simulink model "fuzzyRIP_LQR"  (Simulink 8.1)
settings: Solver=ode45  StartTime=0.0  StopTime=20  RelTol=1e-3
StopFcn:
  | subplot(3,1,1);
  | plot(Data.time, Data.signals(1,1).values,'-r','LineWidth',1.5)
  | legend('alpha');
  | grid;
  | ylabel('alpha [rad]');
  | title ('FuzzyController');
  | subplot(3,1,2);
  | plot(Data.time, Data.signals(1,3).values,'-b','LineWidth',1.5)
  | legend('theta');
  | grid;
  | ylabel('theta [rad]');
  | subplot(3,1,3);
  | plot(Data.time, Data.signals(1,5).values,'-g','LineWidth',1.5)
  | legend('Voltage');
  | grid;
  | ylabel('voltage [V]');
libraries: fuzblock x1
settings Model: Creator=ThanhNhan  LastModifiedBy=ThanhNhan
settings DataIOCC: SignalLoggingSaveFormat=Dataset
settings OptimizationCC: ExpressionDepthLimit=128
settings DebuggingCC: FcnCallInpInsideContextMsg=EnableAllAsError
settings GRTTargetCC: CombineOutputUpdateFcns=on  GRTInterface=off

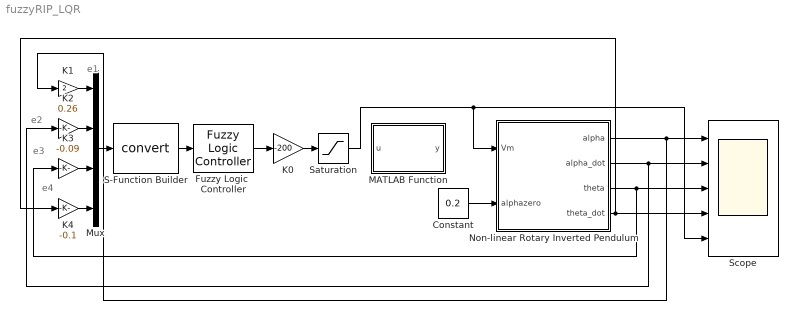
== system fuzzyRIP_LQR ==
  note: e4
  note: e3
  note: e2
  note: e1
  Constant : Constant  Value=0.2
  Fuzzy Logic  Controller : fuzblock/Fuzzy Logic  Controller  fis='RIPfuzzyMam5.fis'
  K0 : Gain  Gain=-200
  K1 : Gain  Gain=2
  K2 : Gain  Gain=0.26
  K3 : Gain  Gain=-0.09
  K4 : Gain  Gain=-0.1
  MATLAB Function : MATLAB Function  TreatAsAtomicUnit=on
  Mux : Mux
  Non-linear Rotary Inverted Pendulum : Subsystem  mask{Jeq=0.004036, g=9.81, m=0.05562, L=0.1254, r=0.1095, Beq=0.0444, eta=0.69, Km=0.084026, Kt=0.084039, Rm=2.6, Jm=0.001}
      mask prompts: Jeq "Momen quán tính tuong duong (Jeq)"; g "Gia toc trong truong (g)"; m "Khoi luong con lac (m)"; L "Nua chieu dai con lac (L)"; r "Nua chieu dài cánh tay (r)"; Beq "He so can tuong duong (Beq)"; eta "Hieu suat dong co (eta)"; Km "Hang so suc dien dong (Km)"; Kt "Hang so momen  (Kt)"; Rm "Dien tro phan ung (Rm)"; Jm "Momen quan tinh dong co (Jm)"
  S-Function Builder : S-Function  InitFcn=try, set_param(gcb,'FunctionName','convert'), end  FunctionName=convert  SFunctionModules=convert_wrapper  WizardData=DataTag0  EnableBusSupport=off  mask(S-Function Builder){}
      mask help: Simulink:masks:SFunctionBuilder_MD
      mask init:
      | val = [[.9  0.75 0.75 1 1 .9 .9 1]',[1 1 0.75 0.75 .9 .9 1 .9]'];try , sys = get_param(gcb,'SfunBuilderFcnName');if isempty(sys), sys = get_param(gcb,'FunctionName'); end,catch, sys = get_param(gcb,'FunctionName'); end
      settings: CopyFcn=set_param(gcbh,'LinkStatus','none')  PreSaveFcn=try, set_param(gcb,'FunctionName','convert'), end  OpenFcn=sfunctionwizard(gcbh)
      mask Display: plot(val(:,1),val(:,2)),disp(sys), port_label('input',1,'u0'), port_label('output',1,'y0')
  Saturation : Saturate  UpperLimit=24  LowerLimit=-24
  Scope : Scope  NumInputPorts=5
      settings: YMin=-29.91~-1500~5e+07~1e+08~-5  YMax=-29.78~1500~4.5e+08~1.1e+09~5  SaveName=Data
  wires:
  Constant/1 -> Non-linear Rotary Inverted Pendulum/2(alphazero)
  Non-linear Rotary Inverted Pendulum/4(theta_dot) -> K4/1, Scope/4
  Non-linear Rotary Inverted Pendulum/3(theta) -> K3/1, Scope/3
  Non-linear Rotary Inverted Pendulum/2(alpha_dot) -> K2/1, Scope/2
  Non-linear Rotary Inverted Pendulum/1(alpha) -> K1/1, Scope/1
  K4/1 -> Mux/4
  K3/1 -> Mux/3
  K2/1 -> Mux/2
  K1/1 -> Mux/1
  Fuzzy Logic  Controller/1 -> K0/1
  K0/1 -> Saturation/1
  S-Function Builder/1 -> Fuzzy Logic  Controller/1
  Mux/1 -> S-Function Builder/1
  Saturation/1 -> Non-linear Rotary Inverted Pendulum/1(Vm), Scope/5

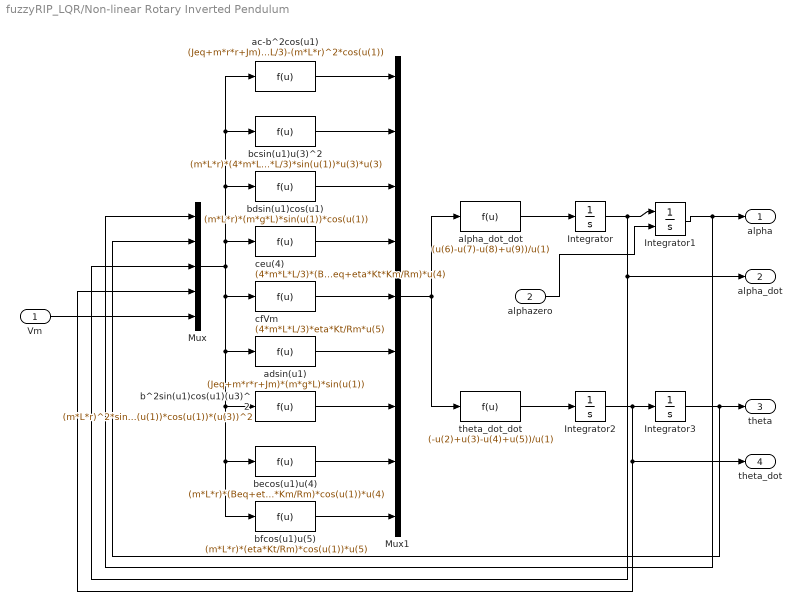
== system fuzzyRIP_LQR/Non-linear Rotary Inverted Pendulum ==
  Vm : Inport
  alphazero : Inport  Port=2
  Integrator : Integrator  UpperSaturationLimit=pi/18  LowerSaturationLimit=-pi/18
  Integrator1 : Integrator  InitialConditionSource=external  UpperSaturationLimit=pi/18  LowerSaturationLimit=-pi/18
  Integrator2 : Integrator
  Integrator3 : Integrator  UpperSaturationLimit=2  LowerSaturationLimit=-2
  Mux : Mux  Inputs=5
  Mux1 : Mux  Inputs=9
  ac-b^2cos(u1) : Fcn  Expr=(Jeq+m*r*r+Jm)*(4*m*L*L/3)-(m*L*r)^2*cos(u(1))
  adsin(u1) : Fcn  Expr=(Jeq+m*r*r+Jm)*(m*g*L)*sin(u(1))
  alpha_dot_dot : Fcn  Expr=(u(6)-u(7)-u(8)+u(9))/u(1)
  b^2sin(u1)cos(u1)(u3)^2 : Fcn  Expr=(m*L*r)^2*sin(u(1))*cos(u(1))*(u(3))^2
  bcsin(u1)u(3)^2 : Fcn  Expr=(m*L*r)*(4*m*L*L/3)*sin(u(1))*u(3)*u(3)
  bdsin(u1)cos(u1) : Fcn  Expr=(m*L*r)*(m*g*L)*sin(u(1))*cos(u(1))
  becos(u1)u(4) : Fcn  Expr=(m*L*r)*(Beq+eta*Kt*Km/Rm)*cos(u(1))*u(4)
  bfcos(u1)u(5) : Fcn  Expr=(m*L*r)*(eta*Kt/Rm)*cos(u(1))*u(5)
  ceu(4) : Fcn  Expr=(4*m*L*L/3)*(Beq+eta*Kt*Km/Rm)*u(4)
  cfVm : Fcn  Expr=(4*m*L*L/3)*eta*Kt/Rm*u(5)
  theta_dot_dot : Fcn  Expr=(-u(2)+u(3)-u(4)+u(5))/u(1)
  alpha : Outport
  alpha_dot : Outport  Port=2
  theta : Outport  Port=3
  theta_dot : Outport  Port=4
  wires:
  alpha_dot_dot/1 -> Integrator/1
  Integrator/1 -> Mux/3, alpha_dot/1, Integrator1/1
  theta_dot_dot/1 -> Integrator2/1
  Integrator1/1 -> Mux/1, alpha/1
  Integrator3/1 -> Mux/2, theta/1
  ac-b^2cos(u1)/1 -> Mux1/1
  bcsin(u1)u(3)^2/1 -> Mux1/2
  bdsin(u1)cos(u1)/1 -> Mux1/3
  ceu(4)/1 -> Mux1/4
  cfVm/1 -> Mux1/5
  adsin(u1)/1 -> Mux1/6
  b^2sin(u1)cos(u1)(u3)^2/1 -> Mux1/7
  becos(u1)u(4)/1 -> Mux1/8
  bfcos(u1)u(5)/1 -> Mux1/9
  Mux1/1 -> theta_dot_dot/1, alpha_dot_dot/1
  Mux/1 -> ceu(4)/1, bdsin(u1)cos(u1)/1, bcsin(u1)u(3)^2/1, ac-b^2cos(u1)/1, bfcos(u1)u(5)/1, becos(u1)u(4)/1, b^2sin(u1)cos(u1)(u3)^2/1, adsin(u1)/1, cfVm/1
  Integrator2/1 -> Mux/4, theta_dot/1, Integrator3/1
  Vm/1 -> Mux/5
  alphazero/1 -> Integrator1/2

== matlab function MATLAB Function ==
  data: u input double; y output double
function y = fcn(u)
%#codegen
if(((0<u)&&(u<0.5))||((0>u)&&(u>-0.5)))
    y=atan(u);
else
y = u;
end
